simulink model "STUDENTS_UAV_SIMULATOR"  (R2021b)
settings: Solver=ode8  StartTime=0.0  StopTime=tf_echelons  FixedStep=0.01  RelTol=1e-4
values from neighbouring files (symbols this model uses):
  initial_pos_conditions = [1 1 0]    [STUDENTS_UAV_SIMULATOR_MAIN.m]
settings Model: Creator=admin  LastModifiedBy=brinonal
settings SolverCC: AlgebraicLoopSolver=TrustRegion
settings DataIOCC: ReturnWorkspaceOutputs=off
settings DebuggingCC: SFMachineParentedDataDiag=warning  ArithmeticOperatorsInVariantConditions=warning
settings SFSimCC: CustomCodeUndefinedFunction=UseInterfaceOnly

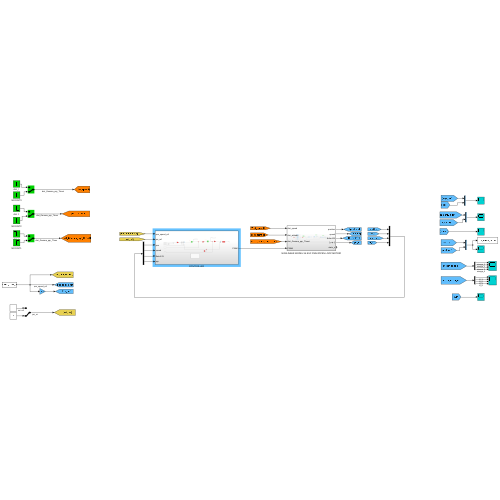
[thumbnail: Simulink's stored preview of the top-level diagram]
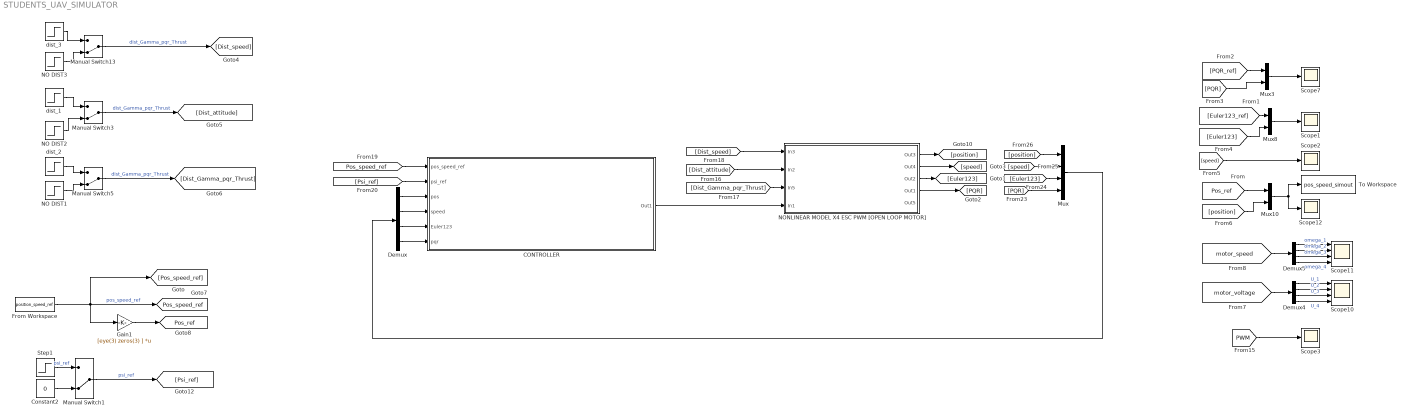
== system STUDENTS_UAV_SIMULATOR ==
  CONTROLLER : Subsystem
  Constant2 : Constant  Value=0
  Demux : Demux
  Demux4 : Demux
  Demux5 : Demux
  From Workspace : FromWorkspace  VariableName=position_speed_ref
  Gain1 : Gain  Gain=[eye(3) zeros(3) ]  Multiplication=Matrix(K*u) (u vector)
  Manual Switch{1,3,5,13} (4 alike) : ManualSwitch  CurrentSetting=0
  Mux : Mux
  Mux10 : Mux  Inputs=2
  Mux3 : Mux  Inputs=2
  Mux8 : Mux  Inputs=2
  NO DIST1 : Step  Time=3  After=[0 0 0 0]
  NO DIST2 : Step  Time=3  After=[0 0 0]
  NO DIST3 : Step  Time=3  After=[0 0 0]
  NONLINEAR MODEL X4 ESC PWM [OPEN LOOP MOTOR] : Subsystem
  Scope{1..3,7,12} (5 alike) : Scope
  Scope10 : Scope  NumInputPorts=4
  Scope11 : Scope  NumInputPorts=4
  Step1 : Step  Time=3  After=0.3  SampleTime=0
  To Workspace : ToWorkspace  VariableName=pos_speed_simout  SaveFormat=Timeseries  SampleTime=-1
  dist_1 : Step  Time=30  After=[-1 0 0]
  dist_2 : Step  Time=30  After=[-1 0 0 0]
  dist_3 : Step  Time=30  After=[-0.3 0 0]
  tag scope: Pos_ref=global, Pos_speed_ref=global
  wires:
  Demux4/3 -> Scope10/3  "U_3"
  NO DIST1/1 -> Manual Switch5/2
  Demux4/4 -> Scope10/4  "U_4"
  dist_1/1 -> Manual Switch3/1
  Demux5/1 -> Scope11/1  "omega_1"
  dist_3/1 -> Manual Switch13/1
  NO DIST3/1 -> Manual Switch13/2
  dist_2/1 -> Manual Switch5/1
  Demux5/2 -> Scope11/2  "omega_2"
  Demux4/1 -> Scope10/1  "U_1"
  Demux4/2 -> Scope10/2  "U_2"
  NO DIST2/1 -> Manual Switch3/2
  Demux5/3 -> Scope11/3  "omega_3"
  Mux10/1 -> To Workspace/1, Scope12/1
  Mux8/1 -> Scope1/1
  Demux5/4 -> Scope11/4  "omega_4"
  Mux3/1 -> Scope7/1
  [Pos_ref] -> Mux10/1
  [Euler123_ref] -> Mux8/1
  [PQR_ref] -> Mux3/1
  Manual Switch5/1 -> [Dist_Gamma_pqr_Thrust]  "dist_Gamma_pqr_Thrust"
  Manual Switch3/1 -> [Dist_attitude]  "dist_Gamma_pqr_Thrust"
  Manual Switch13/1 -> [Dist_speed]  "dist_Gamma_pqr_Thrust"
  [PQR] -> Mux3/2
  [Euler123] -> Mux8/2
  [position] -> Mux10/2
  [speed] -> Scope2/1
  [motor_voltage] -> Demux4/1
  [motor_speed] -> Demux5/1
  [PWM] -> Scope3/1
  [Dist_Gamma_pqr_Thrust] -> NONLINEAR MODEL X4 ESC PWM [OPEN LOOP MOTOR]/3(In5)
  [Dist_attitude] -> NONLINEAR MODEL X4 ESC PWM [OPEN LOOP MOTOR]/2(In2)
  [Dist_speed] -> NONLINEAR MODEL X4 ESC PWM [OPEN LOOP MOTOR]/1(In3)
  Step1/1 -> Manual Switch1/1  "psi_ref"
  [Pos_speed_ref] -> CONTROLLER/1(pos_speed_ref)
  Constant2/1 -> Manual Switch1/2
  Demux/1 -> CONTROLLER/3(pos)
  Demux/2 -> CONTROLLER/4(speed)
  Demux/3 -> CONTROLLER/5(Euler123)
  Demux/4 -> CONTROLLER/6(pqr)
  Mux/1 -> Demux/1
  CONTROLLER/1(Out1) -> NONLINEAR MODEL X4 ESC PWM [OPEN LOOP MOTOR]/4(In1)
  [Psi_ref] -> CONTROLLER/2(psi_ref)
  Manual Switch1/1 -> [Psi_ref]  "psi_ref"
  NONLINEAR MODEL X4 ESC PWM [OPEN LOOP MOTOR]/1(Out3) -> [position]
  NONLINEAR MODEL X4 ESC PWM [OPEN LOOP MOTOR]/2(Out4) -> [speed]
  NONLINEAR MODEL X4 ESC PWM [OPEN LOOP MOTOR]/3(Out2) -> [Euler123]
  NONLINEAR MODEL X4 ESC PWM [OPEN LOOP MOTOR]/4(Out1) -> [PQR]
  [position] -> Mux/1
  [speed] -> Mux/2
  [Euler123] -> Mux/3
  [PQR] -> Mux/4
  Gain1/1 -> [Pos_ref]
  From Workspace/1 -> Gain1/1, [Pos_speed_ref], [Pos_speed_ref]  "pos_speed_ref"

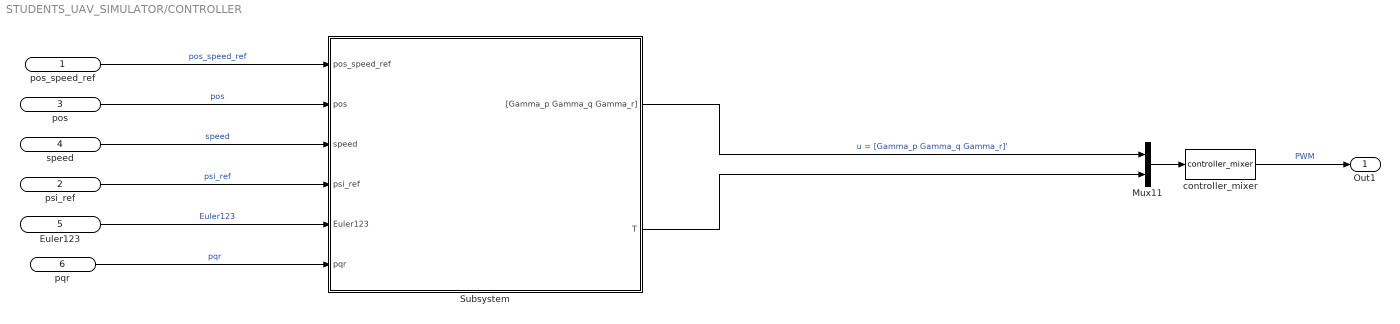
== system STUDENTS_UAV_SIMULATOR/CONTROLLER ==
  pos_speed_ref : Inport
  psi_ref : Inport  Port=2
  pos : Inport  Port=3
  speed : Inport  Port=4
  Euler123 : Inport  Port=5
  pqr : Inport  Port=6
  Mux11 : Mux  Inputs=2
  Subsystem : Subsystem
  "controller_mixer " : MATLABFcn  MATLABFcn=controller_mixer  OutputDimensions=4
  Out1 : Outport  VectorParamsAs1DForOutWhenUnconnected=off
  wires:
  Mux11/1 -> "controller_mixer "/1
  Subsystem/1("[Gamma_p Gamma_q Gamma_r]") -> Mux11/1  "u = [Gamma_p Gamma_q Gamma_r]'"
  "controller_mixer "/1 -> Out1/1  "PWM"
  Subsystem/2(T) -> Mux11/2
  pos_speed_ref/1 -> Subsystem/1(pos_speed_ref)  "pos_speed_ref"
  pos/1 -> Subsystem/2(pos)  "pos"
  speed/1 -> Subsystem/3(speed)  "speed"
  psi_ref/1 -> Subsystem/4(psi_ref)  "psi_ref"
  Euler123/1 -> Subsystem/5(Euler123)  "Euler123"
  pqr/1 -> Subsystem/6(pqr)  "pqr"

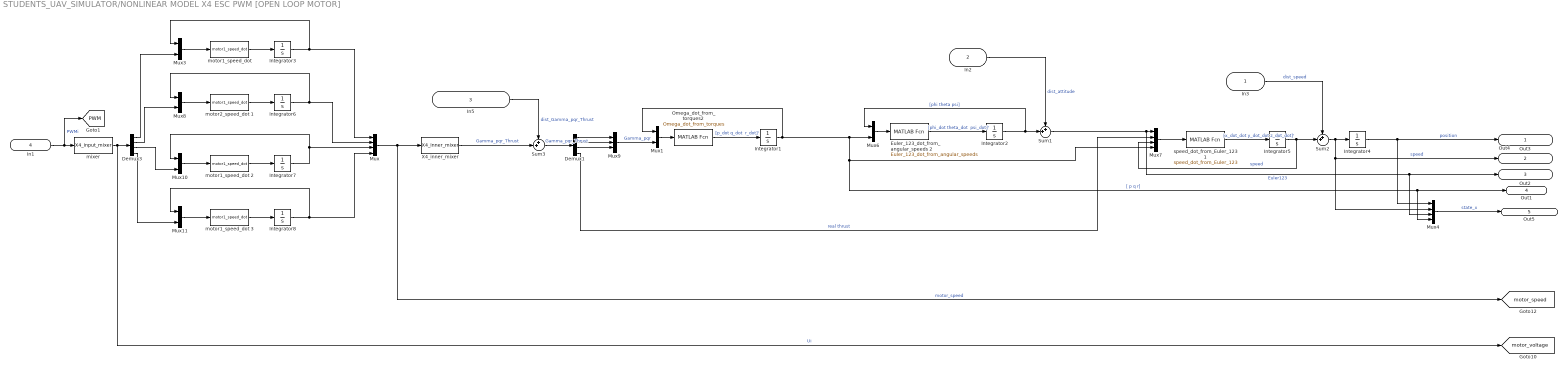
== system STUDENTS_UAV_SIMULATOR/NONLINEAR MODEL X4 ESC PWM [OPEN LOOP MOTOR] ==
  In3 : Inport
  In2 : Inport  Port=2
  In5 : Inport  Port=3
  In1 : Inport  Port=4
  Demux1 : Demux
  Demux3 : Demux
  Euler_123_dot_from_angular_speeds 2 : MATLABFcn  MATLABFcn=Euler_123_dot_from_angular_speeds  OutputDimensions=3
  Integrator1 : Integrator  InitialCondition=[ 0 0 0]
  Integrator{2..3,6..8} (5 alike) : Integrator
  Integrator4 : Integrator  InitialCondition=initial_pos_conditions
  Integrator5 : Integrator  InitialCondition=[0 0 0]
  Mux : Mux
  Mux{1,3,6,8,10..11} (6 alike) : Mux  Inputs=2
  Mux4 : Mux
  Mux7 : Mux
  Mux9 : Mux  Inputs=3
  Omega_dot_from_torques2 : MATLABFcn  MATLABFcn=Omega_dot_from_torques  OutputDimensions=3
  Sum1 : Sum  Inputs=++|
  Sum2 : Sum  Inputs=++|
  Sum3 : Sum  Inputs=++|
  X4_inner_mixer : MATLABFcn  MATLABFcn=X4_inner_mixer  OutputDimensions=4
  "mixer " : MATLABFcn  MATLABFcn=X4_input_mixer  OutputDimensions=4
  "motor1_speed_dot " : MATLABFcn  MATLABFcn=motor1_speed_dot  OutputDimensions=1
  motor1_speed_dot 2 : MATLABFcn  MATLABFcn=motor1_speed_dot  OutputDimensions=1
  motor1_speed_dot 3 : MATLABFcn  MATLABFcn=motor1_speed_dot  OutputDimensions=1
  motor2_speed_dot 1 : MATLABFcn  MATLABFcn=motor1_speed_dot  OutputDimensions=1
  speed_dot_from_Euler_123 1 : MATLABFcn  MATLABFcn=speed_dot_from_Euler_123  OutputDimensions=3
  Out3 : Outport  VectorParamsAs1DForOutWhenUnconnected=off
  Out4 : Outport  Port=2  VectorParamsAs1DForOutWhenUnconnected=off
  Out2 : Outport  Port=3  VectorParamsAs1DForOutWhenUnconnected=off
  Out1 : Outport  Port=4  VectorParamsAs1DForOutWhenUnconnected=off
  Out5 : Outport  Port=5  VectorParamsAs1DForOutWhenUnconnected=off
  tag scope: PWM=global, motor_speed=global, motor_voltage=global
  wires:
  Integrator2/1 -> Sum1/2, Mux6/1  "[phi theta psi]"
  Mux6/1 -> Euler_123_dot_from_angular_speeds 2/1
  Integrator4/1 -> Mux4/1, Out3/1  "position"
  Mux4/1 -> Out5/1  "state_x"
  In3/1 -> Sum2/1  "dist_speed"
  Mux7/1 -> speed_dot_from_Euler_123 1/1
  Integrator5/1 -> Sum2/2, Mux7/3  "speed"
  Integrator1/1 -> Mux6/2, Out1/1, Mux4/4, Mux7/4, Mux1/1  "[ p q r]"
  Demux1/4 -> Mux7/2  "real thrust"
  Demux1/3 -> Mux9/3
  Mux9/1 -> Mux1/2  "Gamma_pqr"
  Demux1/2 -> Mux9/2
  Mux1/1 -> Omega_dot_from_torques2/1
  Demux1/1 -> Mux9/1
  In2/1 -> Sum1/1  "dist_attitude"
  Euler_123_dot_from_angular_speeds 2/1 -> Integrator2/1  "[phi_dot theta_dot  psi_dot]'"
  Omega_dot_from_torques2/1 -> Integrator1/1  "[p_dot q_dot  r_dot]'"
  speed_dot_from_Euler_123 1/1 -> Integrator5/1  "[x_dot_dot y_dot_dot z_dot_dot]'"
  Sum2/1 -> Mux4/2, Out4/1, Integrator4/1  "speed"
  Sum1/1 -> Out2/1, Mux4/3, Mux7/1  "Euler123"
  X4_inner_mixer/1 -> Sum3/2  "Gamma_pqr_Thrust"
  Sum3/1 -> Demux1/1  "Gamma_pqr_Thrust"
  In5/1 -> Sum3/1  "dist_Gamma_pqr_Thrust"
  In1/1 -> [PWM], "mixer "/1  "PWMi"
  "mixer "/1 -> [motor_voltage], Demux3/1  "Ui"
  "motor1_speed_dot "/1 -> Integrator3/1
  Mux3/1 -> "motor1_speed_dot "/1
  Integrator3/1 -> Mux/1, Mux3/1
  Demux3/1 -> Mux3/2
  motor2_speed_dot 1/1 -> Integrator6/1
  Mux8/1 -> motor2_speed_dot 1/1
  Integrator6/1 -> Mux/2, Mux8/1
  Demux3/2 -> Mux8/2
  motor1_speed_dot 2/1 -> Integrator7/1
  Mux10/1 -> motor1_speed_dot 2/1
  Integrator7/1 -> Mux10/1, Mux/3
  motor1_speed_dot 3/1 -> Integrator8/1
  Mux11/1 -> motor1_speed_dot 3/1
  Integrator8/1 -> Mux/4, Mux11/1
  Demux3/3 -> Mux10/2
  Demux3/4 -> Mux11/2
  Mux/1 -> [motor_speed], X4_inner_mixer/1  "motor_speed"

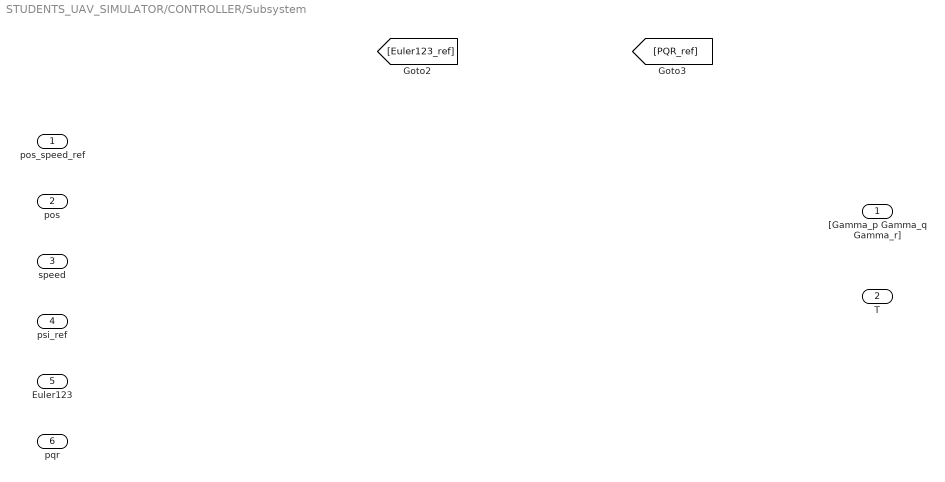
== system STUDENTS_UAV_SIMULATOR/CONTROLLER/Subsystem ==
  pos_speed_ref : Inport
  pos : Inport  Port=2
  speed : Inport  Port=3
  psi_ref : Inport  Port=4
  Euler123 : Inport  Port=5
  pqr : Inport  Port=6
  "[Gamma_p Gamma_q Gamma_r]" : Outport
  T : Outport  Port=2
